simulink model "ASR_ClosedLoop"  (R2019b)
settings: Solver=ode5  StartTime=0.0  StopTime=10  FixedStep=Ts  RelTol=1e-3  EnableMultiTasking=on
values from neighbouring files (symbols this model uses):
  a = 49*cm_unit    (= 0.49)    [ASR_Parameters.m]    (also in System_Trans_Fcn.m)
  b = 27*cm_unit    (= 0.27)    [ASR_Parameters.m]
  dt = Ts    [ASR_Initial_posture.m]    (also in ASR_Parameters.m = 0.05; System_Trans_Fcn.m = 0.05)
  phi_init = deg2rad(65)    [ASR_Initial_posture.m]
  psi_init = deg2rad(5)    [ASR_Initial_posture.m]
  rw = 6.5*cm_unit    (= 0.065)    [ASR_Parameters.m]
  Ts = 5*1e-2    (= 0.05)    [ASR_Parameters.m]
  x_init = [xCr_init;yCr_init;phi_init]    [ASR_Initial_posture.m]
  xCr_init = 0    [ASR_Initial_posture.m]
  yCr_init = 0    [ASR_Initial_posture.m]
undefined symbols (not defined in the file or in its folder): DiscIntNeverNeededParam
libraries: simulink x6, sharedTrackingLibrary x2
settings Model: Creator=nasralla  LastModifiedBy=kerrm
settings SolverCC: AutoInsertRateTranBlk=on
settings DataIOCC: SaveFormat=Array  SignalLoggingSaveFormat=ModelDataLogs  ReturnWorkspaceOutputs=off
settings OptimizationCC: ExpressionDepthLimit=2147483647  InitFltsAndDblsToZero=on  LifeSpan=inf
settings DebuggingCC: SaveWithParameterizedLinksMsg=none  UnderspecifiedInitializationDetection=Classic  MergeDetectMultiDrivingBlocksExec=none  SolverPrmCheckMsg=warning  FcnCallInpInsideContextMsg=warning  StateNameClashWarn=warning  SFUnexpectedBacktrackingDiag=warning  SFNoUnconditionalDefaultTransitionDiag=warning  SFExecutionAtInitializationDiag=none  ArithmeticOperatorsInVariantConditions=warning
settings HardwareCC: ProdBitPerPointer=32  ProdBitPerSizeT=32  ProdBitPerPtrDiffT=32  ProdLargestAtomicFloat=None  ProdIntDivRoundTo=Undefined  ProdEndianess=Unspecified  ProdWordSize=32  ProdHWDeviceType=32-bit Generic
settings ModelReferenceCC: PropagateSignalLabelsOutOfModel=off
settings SFSimCC: SimUseLocalCustomCode=off  CustomCodeUndefinedFunction=UseInterfaceOnly
settings RTWCC: RTWUseLocalCustomCode=off
settings CodeAppCC: StateflowObjectComments=on
settings GRTTargetCC: TargetFcnLib=ansi_tfl_tmw.mat  TargetLangStandard=C89/C90 (ANSI)  CombineOutputUpdateFcns=off  GRTInterface=on
settings ConfigComp: CovMetricSettings=dw  CovHtmlReporting=on  CovSaveCumulativeToWorkspaceVar=on  CovSaveSingleToWorkspaceVar=on  CovExternalEMLEnable=off

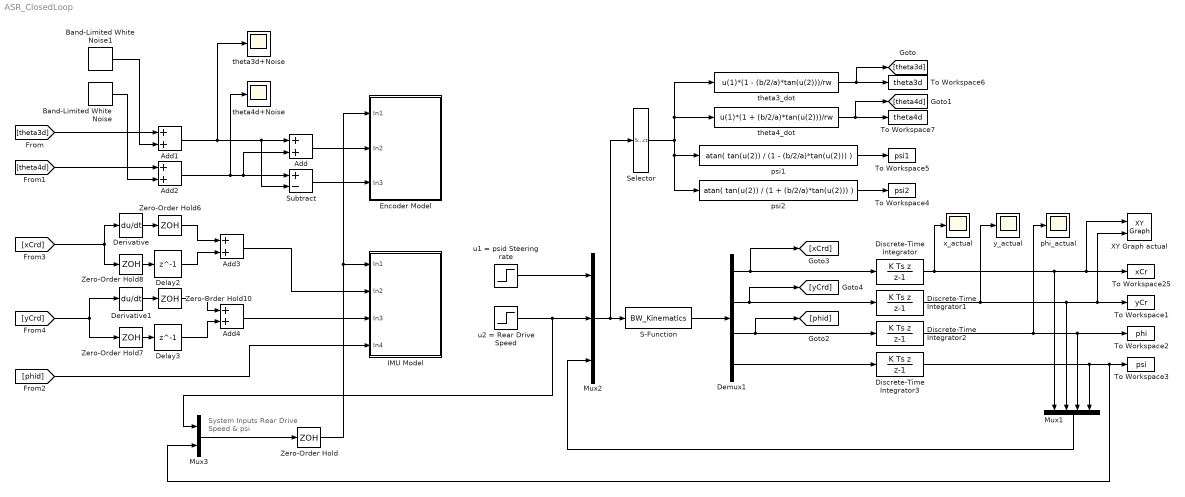
== system ASR_ClosedLoop ==
  note: System Inputs
      | Rear Drive Speed  & psi
  Add{,1..4} (5 alike) : Sum
  Band-Limited White Noise : simulink/Sources/Band-Limited White Noise  Cov=[0.1]  Ts=0.1  seed=[23341]
  Band-Limited White Noise1 : simulink/Sources/Band-Limited White Noise  Cov=[0.5]  Ts=0.1  seed=[23341]
  Delay2 : Delay  DelayLength=1  InitialCondition=0  UseCircularBuffer=on
  Delay3 : Delay  DelayLength=1  InitialCondition=0  UseCircularBuffer=on
  Demux1 : Demux
  Derivative : Derivative
  Derivative1 : Derivative
  Discrete-Time Integrator : DiscreteIntegrator  IntegratorMethod=Integration: Backward Euler  InitialCondition=xCr_init  SampleTime=-1  ICPrevOutput=DiscIntNeverNeededParam  ICPrevScaledInput=DiscIntNeverNeededParam
  Discrete-Time Integrator1 : DiscreteIntegrator  IntegratorMethod=Integration: Backward Euler  InitialCondition=yCr_init  SampleTime=-1  ICPrevOutput=DiscIntNeverNeededParam  ICPrevScaledInput=DiscIntNeverNeededParam
  Discrete-Time Integrator2 : DiscreteIntegrator  IntegratorMethod=Integration: Backward Euler  InitialCondition=phi_init  SampleTime=-1  ICPrevOutput=DiscIntNeverNeededParam  ICPrevScaledInput=DiscIntNeverNeededParam
  Discrete-Time Integrator3 : DiscreteIntegrator  IntegratorMethod=Integration: Backward Euler  InitialCondition=psi_init  SampleTime=-1  ICPrevOutput=DiscIntNeverNeededParam  ICPrevScaledInput=DiscIntNeverNeededParam
  Encoder Model : Subsystem
  IMU Model : Subsystem
  Mux1 : Mux
  Mux2 : Mux  Inputs=3
  Mux3 : Mux  Inputs=2
  S-Function : S-Function  FunctionName=BW_Kinematics  SFunctionDeploymentMode=off  EnableBusSupport=off
  Selector : Selector  InputPortWidth=6  IndexOptions=Index vector (dialog)  Indices=[2 6]  OutputSizes=1
  Subtract : Sum  Inputs=+-
  To Workspace1 : ToWorkspace  VariableName=yCr  SampleTime=-1
  To Workspace2 : ToWorkspace  VariableName=phi  SampleTime=-1
  To Workspace25 : ToWorkspace  VariableName=xCr  SampleTime=-1
  To Workspace3 : ToWorkspace  VariableName=psi  SampleTime=-1
  To Workspace4 : ToWorkspace  VariableName=psi2  SampleTime=-1
  To Workspace5 : ToWorkspace  VariableName=psi1  SampleTime=-1
  To Workspace6 : ToWorkspace  VariableName=theta3d  SampleTime=-1
  To Workspace7 : ToWorkspace  VariableName=theta4d  SampleTime=-1
  XY Graph actual : simulink/Sinks/XY Graph  xmin=-1  xmax=5  ymin=-1  ymax=5  st=-1
  Zero-Order Hold{,6..8,10} (5 alike) : ZeroOrderHold  SampleTime=Ts
  phi_actual : Scope
  psi1 : Fcn  Expr=atan( tan(u(2)) / (1 - (b/2/a)*tan(u(2))) )
  psi2 : Fcn  Expr=atan( tan(u(2)) / (1 + (b/2/a)*tan(u(2))) )
  theta3_dot : Fcn  Expr=u(1)*(1 - (b/2/a)*tan(u(2)))/rw
  theta3d+Noise : Scope
  theta4_dot : Fcn  Expr=u(1)*(1 + (b/2/a)*tan(u(2)))/rw
  theta4d+Noise : Scope
  u1 = psid Steering rate : Step  Time=3  After=0  SampleTime=0
  u2 = Rear Drive Speed : Step  Time=0  After=.5  SampleTime=0
  x_actual : Scope
  y_actual : Scope
  wires:
  S-Function/1 -> Demux1/1
  Mux2/1 -> Selector/1, S-Function/1
  Mux1/1 -> Mux2/3
  Selector/1 -> psi2/1, psi1/1, theta4_dot/1, theta3_dot/1
  psi2/1 -> To Workspace4/1
  psi1/1 -> To Workspace5/1
  theta4_dot/1 -> [theta4d], To Workspace7/1
  theta3_dot/1 -> [theta3d], To Workspace6/1
  Discrete-Time Integrator3/1 -> Mux3/2, To Workspace3/1, Mux1/4
  Discrete-Time Integrator/1 -> XY Graph actual/1, To Workspace25/1, Mux1/1, x_actual/1
  Demux1/1 -> Discrete-Time Integrator/1, [xCrd]
  Discrete-Time Integrator1/1 -> XY Graph actual/2, To Workspace1/1, Mux1/2, y_actual/1
  Demux1/2 -> [yCrd], Discrete-Time Integrator1/1
  Discrete-Time Integrator2/1 -> Mux1/3, To Workspace2/1, phi_actual/1
  Demux1/3 -> [phid], Discrete-Time Integrator2/1
  Demux1/4 -> Discrete-Time Integrator3/1
  Mux3/1 -> Zero-Order Hold/1
  Zero-Order Hold/1 -> IMU Model/1(In1), Encoder Model/1(In1)
  [theta3d] -> Add1/1
  Add1/1 -> theta3d+Noise/1, Add/1, Subtract/2
  [theta4d] -> Add2/1
  Add2/1 -> Subtract/1, Add/2, theta4d+Noise/1
  u2 = Rear Drive Speed/1 -> Mux3/1, Mux2/2
  u1 = psid Steering rate/1 -> Mux2/1
  Zero-Order Hold7/1 -> Delay3/1
  [xCrd] -> Derivative/1, Zero-Order Hold8/1
  [yCrd] -> Derivative1/1, Zero-Order Hold7/1
  Derivative1/1 -> Zero-Order Hold10/1
  Delay3/1 -> Add4/2
  Derivative/1 -> Zero-Order Hold6/1
  Zero-Order Hold6/1 -> Add3/1
  Zero-Order Hold10/1 -> Add4/1
  Band-Limited White Noise/1 -> Add2/2
  Band-Limited White Noise1/1 -> Add1/2
  Delay2/1 -> Add3/2
  Zero-Order Hold8/1 -> Delay2/1
  Add3/1 -> IMU Model/2(In2)
  Add4/1 -> IMU Model/3(In3)
  [phid] -> IMU Model/4(In4)
  Add/1 -> Encoder Model/2(In2)
  Subtract/1 -> Encoder Model/3(In3)

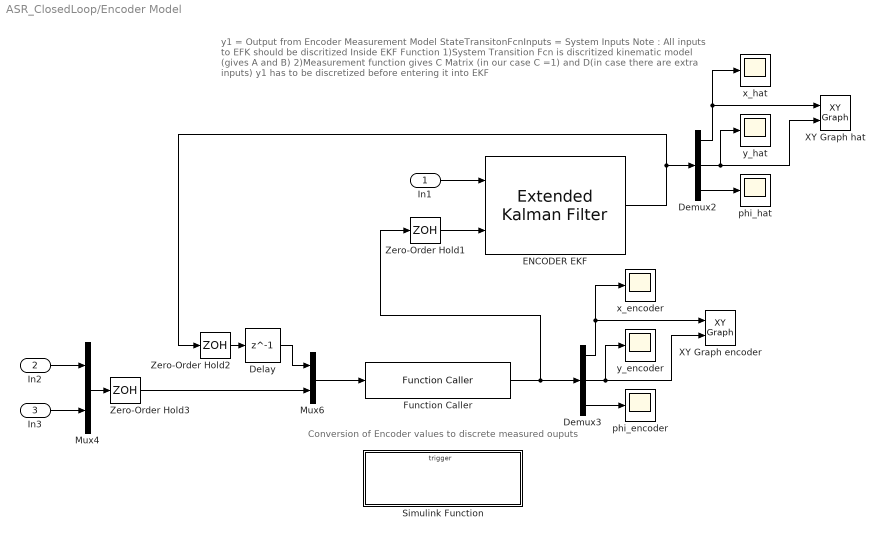
== system ASR_ClosedLoop/Encoder Model ==
  note: Conversion of Encoder values to discrete measured ouputs
  note: y1 = Output from Encoder Measurement Model
      | StateTransitonFcnInputs = System Inputs
      | Note : All inputs to EFK should be discritized
      | Inside EKF Function
      | 1)System Transition Fcn is discritized kinematic model (gives A and B)
      | 2)Measurement function gives C Matrix (in our case C =1) and D(in case there are extra inputs)
      | y1 has to be discretized before entering it into EKF
  In1 : Inport
  In2 : Inport  Port=2
  In3 : Inport  Port=3
  Delay : Delay  DelayLength=1  InitialCondition=x_init  UseCircularBuffer=on
  Demux2 : Demux  Outputs=3
  Demux3 : Demux  Outputs=3
  ENCODER EKF : sharedTrackingLibrary/Extended Kalman Filter  StateTransitionFcn=System_Trans_Fcn  HasStateTransitionJacobianFcn=off  HasAdditiveProcessNoise=Additive  ProcessNoise=Q_E  HasTimeVaryingProcessNoise=off  HasStateTransitionFcnExtraArgument=1  InitialState=x_init  InitialStateCovariance=P_init_E  MeasurementFcn1=ASR_Measurement  HasMeasurementJacobianFcn1=off  HasMeasurementEnablePort1=off  HasAdditiveMeasurementNoise1=Additive  MeasurementNoise1=R_E  HasTimeVaryingMeasurementNoise1=off  HasMeasurementFcnExtraArgument1=0  MeasurementFcn2=myMeasurementFcn  HasMeasurementJacobianFcn2=off  HasMeasurementEnablePort2=off  HasAdditiveMeasurementNoise2=Additive  MeasurementNoise2=1  HasTimeVaryingMeasurementNoise2=off  HasMeasurementFcnExtraArgument2=0  MeasurementFcn3=myMeasurementFcn  HasMeasurementJacobianFcn3=off  HasMeasurementEnablePort3=off  HasAdditiveMeasurementNoise3=Additive  MeasurementNoise3=1  HasTimeVaryingMeasurementNoise3=off  HasMeasurementFcnExtraArgument3=0  MeasurementFcn4=myMeasurementFcn  HasMeasurementJacobianFcn4=off  HasMeasurementEnablePort4=off  HasAdditiveMeasurementNoise4=Additive  MeasurementNoise4=1  HasTimeVaryingMeasurementNoise4=off  HasMeasurementFcnExtraArgument4=0  MeasurementFcn5=myMeasurementFcn  HasMeasurementJacobianFcn5=off  HasMeasurementEnablePort5=off  HasAdditiveMeasurementNoise5=Additive  MeasurementNoise5=1  HasTimeVaryingMeasurementNoise5=off  HasMeasurementFcnExtraArgument5=0  EnableMultirate=off  StateTransitionFcnSampleTime=1  MeasurementFcn1SampleTime=1  MeasurementFcn2SampleTime=1  MeasurementFcn3SampleTime=1  MeasurementFcn4SampleTime=1  MeasurementFcn5SampleTime=1  UseCurrentEstimator=on  OutputStateCovariance=off  DataType=double  SampleTime=Ts  NumberOfMeasurements=1
      settings: SourceProductName=Automated Driving Toolbox  SourceProductBaseCode=DR
  Function Caller : FunctionCaller  FunctionPrototype=y = encoder_measurement(u)  InputArgumentSpecifications=<Enter example>  OutputArgumentSpecifications=<Enter example>
  Mux4 : Mux  Inputs=2
  Mux6 : Mux  Inputs=2
  Simulink Function : Subsystem  TreatAsAtomicUnit=on
  XY Graph encoder : simulink/Sinks/XY Graph  xmin=-1  xmax=5  ymin=-1  ymax=5  st=-1
  XY Graph hat : simulink/Sinks/XY Graph  xmin=-1  xmax=5  ymin=-1  ymax=5  st=-1
  Zero-Order Hold1 : ZeroOrderHold  SampleTime=Ts
  Zero-Order Hold2 : ZeroOrderHold  SampleTime=Ts
  Zero-Order Hold3 : ZeroOrderHold  SampleTime=Ts
  phi_encoder : Scope
  phi_hat : Scope
  x_encoder : Scope
  x_hat : Scope
  y_encoder : Scope
  y_hat : Scope
  wires:
  Zero-Order Hold3/1 -> Mux6/2
  Demux2/3 -> phi_hat/1
  Demux2/2 -> XY Graph hat/2, y_hat/1
  In1/1 -> ENCODER EKF/1
  Demux2/1 -> XY Graph hat/1, x_hat/1
  Demux3/3 -> phi_encoder/1
  Demux3/1 -> x_encoder/1, XY Graph encoder/1
  Zero-Order Hold2/1 -> Delay/1
  Delay/1 -> Mux6/1
  ENCODER EKF/1 -> Demux2/1, Zero-Order Hold2/1
  Mux4/1 -> Zero-Order Hold3/1
  Zero-Order Hold1/1 -> ENCODER EKF/2
  Function Caller/1 -> Zero-Order Hold1/1, Demux3/1
  Mux6/1 -> Function Caller/1
  Demux3/2 -> XY Graph encoder/2, y_encoder/1
  In3/1 -> Mux4/2
  In2/1 -> Mux4/1

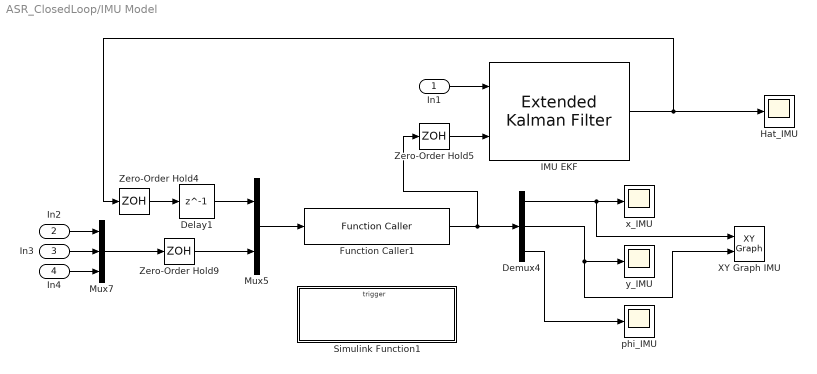
== system ASR_ClosedLoop/IMU Model ==
  In1 : Inport
  In2 : Inport  Port=2
  In3 : Inport  Port=3
  In4 : Inport  Port=4
  Delay1 : Delay  DelayLength=1  InitialCondition=x_init  UseCircularBuffer=on
  Demux4 : Demux  Outputs=3
  Function Caller1 : FunctionCaller  FunctionPrototype=y = IMU_measurement(u)  InputArgumentSpecifications=<Enter example>  OutputArgumentSpecifications=<Enter example>
  Hat_IMU : Scope
  IMU EKF : sharedTrackingLibrary/Extended Kalman Filter  StateTransitionFcn=System_Trans_Fcn  HasStateTransitionJacobianFcn=off  HasAdditiveProcessNoise=Additive  ProcessNoise=Q_IMU  HasTimeVaryingProcessNoise=off  HasStateTransitionFcnExtraArgument=1  InitialState=x_init  InitialStateCovariance=P_init_IMU  MeasurementFcn1=ASR_Measurement  HasMeasurementJacobianFcn1=off  HasMeasurementEnablePort1=off  HasAdditiveMeasurementNoise1=Additive  MeasurementNoise1=R_IMU  HasTimeVaryingMeasurementNoise1=off  HasMeasurementFcnExtraArgument1=0  MeasurementFcn2=myMeasurementFcn  HasMeasurementJacobianFcn2=off  HasMeasurementEnablePort2=off  HasAdditiveMeasurementNoise2=Additive  MeasurementNoise2=1  HasTimeVaryingMeasurementNoise2=off  HasMeasurementFcnExtraArgument2=0  MeasurementFcn3=myMeasurementFcn  HasMeasurementJacobianFcn3=off  HasMeasurementEnablePort3=off  HasAdditiveMeasurementNoise3=Additive  MeasurementNoise3=1  HasTimeVaryingMeasurementNoise3=off  HasMeasurementFcnExtraArgument3=0  MeasurementFcn4=myMeasurementFcn  HasMeasurementJacobianFcn4=off  HasMeasurementEnablePort4=off  HasAdditiveMeasurementNoise4=Additive  MeasurementNoise4=1  HasTimeVaryingMeasurementNoise4=off  HasMeasurementFcnExtraArgument4=0  MeasurementFcn5=myMeasurementFcn  HasMeasurementJacobianFcn5=off  HasMeasurementEnablePort5=off  HasAdditiveMeasurementNoise5=Additive  MeasurementNoise5=1  HasTimeVaryingMeasurementNoise5=off  HasMeasurementFcnExtraArgument5=0  EnableMultirate=off  StateTransitionFcnSampleTime=1  MeasurementFcn1SampleTime=1  MeasurementFcn2SampleTime=1  MeasurementFcn3SampleTime=1  MeasurementFcn4SampleTime=1  MeasurementFcn5SampleTime=1  UseCurrentEstimator=on  OutputStateCovariance=off  DataType=double  SampleTime=Ts  NumberOfMeasurements=1
      settings: SourceProductName=Automated Driving Toolbox  SourceProductBaseCode=DR
  Mux5 : Mux  Inputs=2
  Mux7 : Mux  Inputs=3
  Simulink Function1 : Subsystem  TreatAsAtomicUnit=on
  XY Graph IMU : simulink/Sinks/XY Graph  xmin=-1  xmax=5  ymin=-1  ymax=5  st=-1
  Zero-Order Hold4 : ZeroOrderHold  SampleTime=Ts
  Zero-Order Hold5 : ZeroOrderHold  SampleTime=Ts
  Zero-Order Hold9 : ZeroOrderHold  SampleTime=Ts
  phi_IMU : Scope
  x_IMU : Scope
  y_IMU : Scope
  wires:
  Demux4/3 -> phi_IMU/1
  IMU EKF/1 -> Hat_IMU/1, Zero-Order Hold4/1
  Delay1/1 -> Mux5/1
  Demux4/2 -> XY Graph IMU/2, y_IMU/1
  Mux5/1 -> Function Caller1/1
  Function Caller1/1 -> Zero-Order Hold5/1, Demux4/1
  Zero-Order Hold9/1 -> Mux5/2
  In1/1 -> IMU EKF/1
  Demux4/1 -> x_IMU/1, XY Graph IMU/1
  In2/1 -> Mux7/1
  Zero-Order Hold5/1 -> IMU EKF/2
  Mux7/1 -> Zero-Order Hold9/1
  Zero-Order Hold4/1 -> Delay1/1
  In4/1 -> Mux7/3
  In3/1 -> Mux7/2

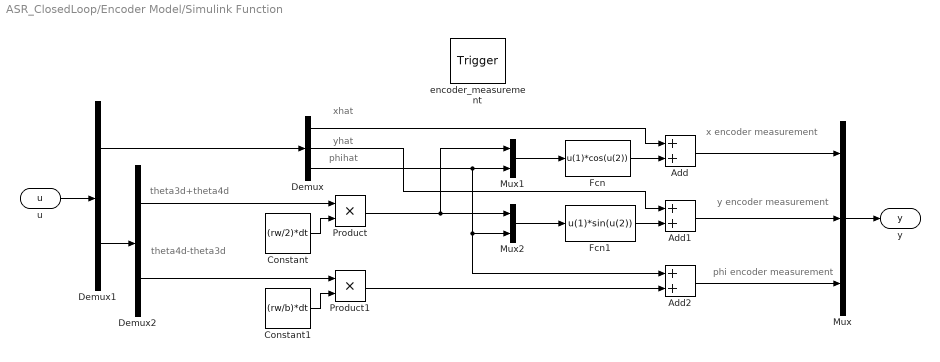
== system ASR_ClosedLoop/Encoder Model/Simulink Function ==
  note: x encoder measurement
  note: theta3d+theta4d
  note: phihat
  note: yhat
  note: xhat
  note: theta4d-theta3d
  note: y encoder measurement
  note: phi encoder measurement
  encoder_measurement : TriggerPort  TriggerType=function-call  IsSimulinkFunction=on  FunctionName=encoder_measurement  FunctionVisibility=scoped  VariantControl=(inherit)
  Add : Sum
  Add1 : Sum
  Add2 : Sum
  Constant : Constant  Value=(rw/2)*dt
  Constant1 : Constant  Value=(rw/b)*dt
  Demux : Demux  Outputs=3
  Demux1 : Demux  Outputs=2
  Demux2 : Demux  Outputs=2
  Fcn : Fcn  Expr=u(1)*cos(u(2))
  Fcn1 : Fcn  Expr=u(1)*sin(u(2))
  Mux : Mux  Inputs=3
  Mux1 : Mux  Inputs=2
  Mux2 : Mux  Inputs=2
  Product : Product
  Product1 : Product
  u : ArgIn  DisableCoverage=on  PortDimensions=5  ArgumentName=u
  y : ArgOut  DisableCoverage=on  PortDimensions=3  ArgumentName=y
  wires:
  u/1 -> Demux1/1
  Demux1/1 -> Demux/1
  Demux1/2 -> Demux2/1
  Demux/1 -> Add/1
  Demux2/1 -> Product/1
  Demux/2 -> Add1/1
  Demux/3 -> Mux1/2, Mux2/2, Add2/1
  Demux2/2 -> Product1/1
  Product1/1 -> Add2/2
  Mux/1 -> y/1
  Constant/1 -> Product/2
  Constant1/1 -> Product1/2
  Product/1 -> Mux1/1, Mux2/1
  Mux1/1 -> Fcn/1
  Mux2/1 -> Fcn1/1
  Fcn/1 -> Add/2
  Fcn1/1 -> Add1/2
  Add/1 -> Mux/1
  Add1/1 -> Mux/2
  Add2/1 -> Mux/3

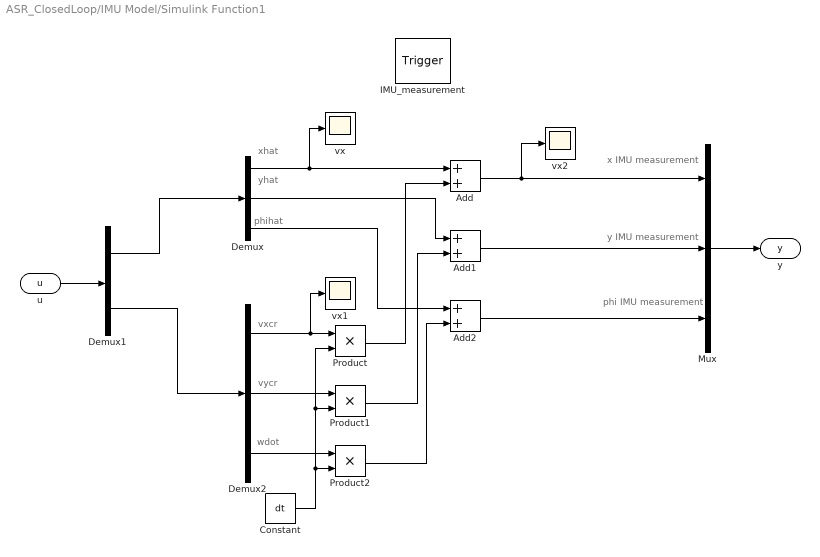
== system ASR_ClosedLoop/IMU Model/Simulink Function1 ==
  note: x IMU measurement
  note: vxcr
  note: phihat
  note: yhat
  note: xhat
  note: vycr
  note: y IMU measurement
  note: phi IMU measurement
  note: wdot
  IMU_measurement : TriggerPort  TriggerType=function-call  IsSimulinkFunction=on  FunctionName=IMU_measurement  FunctionVisibility=scoped  VariantControl=(inherit)
  Add : Sum
  Add1 : Sum
  Add2 : Sum
  Constant : Constant  Value=dt
  Demux : Demux  Outputs=3
  Demux1 : Demux  Outputs=2
  Demux2 : Demux  Outputs=3
  Mux : Mux  Inputs=3
  Product : Product
  Product1 : Product
  Product2 : Product
  vx : Scope
  vx1 : Scope
  vx2 : Scope
  u : ArgIn  DisableCoverage=on  PortDimensions=6  ArgumentName=u
  y : ArgOut  DisableCoverage=on  PortDimensions=3  ArgumentName=y
  wires:
  u/1 -> Demux1/1
  Demux1/1 -> Demux/1
  Demux1/2 -> Demux2/1
  Mux/1 -> y/1
  Add/1 -> Mux/1, vx2/1
  Add1/1 -> Mux/2
  Demux/1 -> vx/1, Add/1
  Demux2/1 -> Product/1, vx1/1
  Demux/2 -> Add1/1
  Demux2/2 -> Product1/1
  Demux/3 -> Add2/1
  Add2/1 -> Mux/3
  Demux2/3 -> Product2/1
  Constant/1 -> Product1/2, Product/2, Product2/2
  Product2/1 -> Add2/2
  Product1/1 -> Add1/2
  Product/1 -> Add/2
